simulink model "Demo_veDYNA_cs"  (Simulink 7.6)
settings: Solver=ode1  SolverMode=SingleTasking  StartTime=0  StopTime=15  FixedStep=1/500  RelTol=1e-3
PreLoadFcn:
  | PreScanveDYNAPreLoadFcn(bdroot);
  | check_NUTS_defined;
  | 
  | assignin('base',['model_closed_' bdroot],false);
PostLoadFcn:
  | PreScanveDYNAPostLoadFcn(bdroot);
  | 
InitFcn:
  | vdy_SetExternalInputSource('ManLongCtrl',1,'Brake','other');
  | vdy_SetExternalInputSource('ManLongCtrl',1,'EngineTorque','other');
  | vdy_SetExternalInputSource('ManLatCtrl',1,'Steering','other');
  | 
  | PreScanveDYNAInitFcn(bdroot);
  | PreScanExperimentInitFcn(bdroot)
StopFcn:
  | PreScanExperimentStopFcn(bdroot)
undefined symbols (not defined in the file): at_period, CPT, DiscIntNeverNeededParam, vm_at_pulsewidth, vm_driver_dflt_gain, x_ini_VRML, y_ini_VRML, z_ini_VRML
libraries: dyna_cpt_lib x93, PreScanSimulinkLibrary x10, PreScanUsefulBlocks x4, simulink x4, anilib x3, dyna_lib x3, simulink_extras x2, dyna_manctrl_lib x2, dyna_road_lib x2, dyna_io_lib x1, dyna_demo_lib x1, dyna_usr_maneuver_states_lib x1
(part 4 of 8)

== system Demo_veDYNA_cs/Mazda_RX8_1/AIR_1_Demux/Signal2ArrayOfSignals5 ==
  note: Set mask parameter VECTORLENGTH
      |  to MAXMESSAGES
  note: Initial state of Previous vector block
      | set to zeros(VECTORLENGTH,1)
  LoopIndex : Inport
  Element : Inport  Port=2
  Assignment : Assignment  IndexOptions=Index vector (port)  Indices=1  OutputSizes=1
  Previous vector : Memory  X0=zeros(VECTORLENGTH,1)  InheritSampleTime=on
  ArrayofElements : Outport
  wires:
  Element/1 -> Assignment/2
  LoopIndex/1 -> Assignment/3
  Previous vector/1 -> Assignment/1
  Assignment/1 -> ArrayofElements/1, Previous vector/1

== system Demo_veDYNA_cs/Mazda_RX8_1/AIR_1_Demux/Signal2ArrayOfSignals6 ==
  note: Set mask parameter VECTORLENGTH
      |  to MAXMESSAGES
  note: Initial state of Previous vector block
      | set to zeros(VECTORLENGTH,1)
  LoopIndex : Inport
  Element : Inport  Port=2
  Assignment : Assignment  IndexOptions=Index vector (port)  Indices=1  OutputSizes=1
  Previous vector : Memory  X0=zeros(VECTORLENGTH,1)  InheritSampleTime=on
  ArrayofElements : Outport
  wires:
  Element/1 -> Assignment/2
  LoopIndex/1 -> Assignment/3
  Previous vector/1 -> Assignment/1
  Assignment/1 -> ArrayofElements/1, Previous vector/1

== system Demo_veDYNA_cs/Mazda_RX8_1/SELF_Demux/compas converter ==
  rotz [rad] : Inport
  cart2compas : Subsystem
  rad2deg : Gain  Gain=180/pi
  heading [deg] : Outport
  wires:
  cart2compas/1(heading [deg]) -> heading [deg]/1
  rotz [rad]/1 -> rad2deg/1
  rad2deg/1 -> cart2compas/1(Angle [deg])

== system Demo_veDYNA_cs/Mazda_RX8_1/Simple ACC/Delta control ==
  R : Inport
  theta : Inport  Port=2
  y_dist : Inport  Port=3
  Add : Sum  Inputs=+-
  Complex to Magnitude-Angle1 : ComplexToMagnitudeAngle
  Polar2Cart : Subsystem
  Real-Imag to Complex1 : RealImagToComplex
  Selector : Selector  IndexOptions=Index vector (dialog)  Indices=[1]  OutputSizes=1
  Terminator_1 : Terminator
  delta gain : Gain  Gain=50  SaturateOnIntegerOverflow=on  OutDataTypeStr=Inherit: Same as input  ParamDataTypeStr=Inherit: Same as input
  preview_distance : Constant  Value=2
  delta : Outport
  wires:
  Selector/1 -> Polar2Cart/2(theta)
  theta/1 -> Selector/1
  R/1 -> Polar2Cart/1(R)
  Polar2Cart/1(y) -> Add/1  "yrel"
  Complex to Magnitude-Angle1/1 -> Terminator_1/1
  delta gain/1 -> delta/1
  preview_distance/1 -> Real-Imag to Complex1/1
  Add/1 -> Real-Imag to Complex1/2
  y_dist/1 -> Add/2
  Real-Imag to Complex1/1 -> Complex to Magnitude-Angle1/1
  Complex to Magnitude-Angle1/2 -> delta gain/1

== system Demo_veDYNA_cs/Mazda_RX8_1/Simple ACC/Engine Torque Control ==
  dist Traffic : Inport
  Vehicle Info : Inport  Port=2
  vSoll : Inport  Port=3
  Brake gain : Gain  Gain=60
  Demux Vehicle Info : Subsystem
  Distance Control : Subsystem  TreatAsAtomicUnit=on
  MinMax : MinMax  Inputs=2  SaturateOnIntegerOverflow=on  InputSameDT=on
  Speed Control : Subsystem  TreatAsAtomicUnit=on
  Brake Pedal : Outport
  Engine Torque : Outport  Port=2
  wires:
  Brake gain/1 -> Brake Pedal/1
  Distance Control/2(Brake Pedal) -> Brake gain/1
  Demux Vehicle Info/4(mmot_diff) -> Speed Control/3(mmot_diff)
  Demux Vehicle Info/3(v_akt1) -> Distance Control/3(v_akt)
  vSoll/1 -> Demux Vehicle Info/2(vSoll)
  Demux Vehicle Info/2(mmot_MIN) -> Speed Control/2(mmot_MIN), Distance Control/2(mmot_MIN)
  Demux Vehicle Info/1(mmot_MAX) -> Distance Control/1(mmot_MAX), Speed Control/1(mmot_MAX)
  MinMax/1 -> Engine Torque/1
  Distance Control/1(Engine Torque) -> MinMax/2
  Speed Control/1(Engine Torque) -> MinMax/1
  dist Traffic/1 -> Distance Control/4(s_diff)
  Vehicle Info/1 -> Demux Vehicle Info/1(Vehicle Info)

== system Demo_veDYNA_cs/Nissan_Cabstar_1/SELF_Demux/compas converter ==
  rotz [rad] : Inport
  cart2compas : Subsystem
  rad2deg : Gain  Gain=180/pi
  heading [deg] : Outport
  wires:
  cart2compas/1(heading [deg]) -> heading [deg]/1
  rotz [rad]/1 -> rad2deg/1
  rad2deg/1 -> cart2compas/1(Angle [deg])

== system Demo_veDYNA_cs/Nissan_Cabstar_1/Trajectories/PathFollowerSva_2 ==
  From Workspace : FromWorkspace  VariableName=trajectory  SampleTime=TimeStep  OutputAfterFinalValue=Holding final value
  From Workspace1 : FromWorkspace  VariableName=trajectory  SampleTime=TimeStep  OutputAfterFinalValue=Setting to zero
  Mux : Mux  Inputs=2
  Selector1 : Selector  InputPortWidth=24  IndexOptions=Index vector (dialog)  Indices=[7:18]  OutputSizes=1
  Selector9 : Selector  InputPortWidth=24  IndexOptions=Index vector (dialog)  Indices=[1:6]  OutputSizes=1
  trajectory : Outport
  wires:
  Selector1/1 -> Mux/2
  Selector9/1 -> Mux/1
  Mux/1 -> trajectory/1
  From Workspace1/1 -> Selector1/1
  From Workspace/1 -> Selector9/1

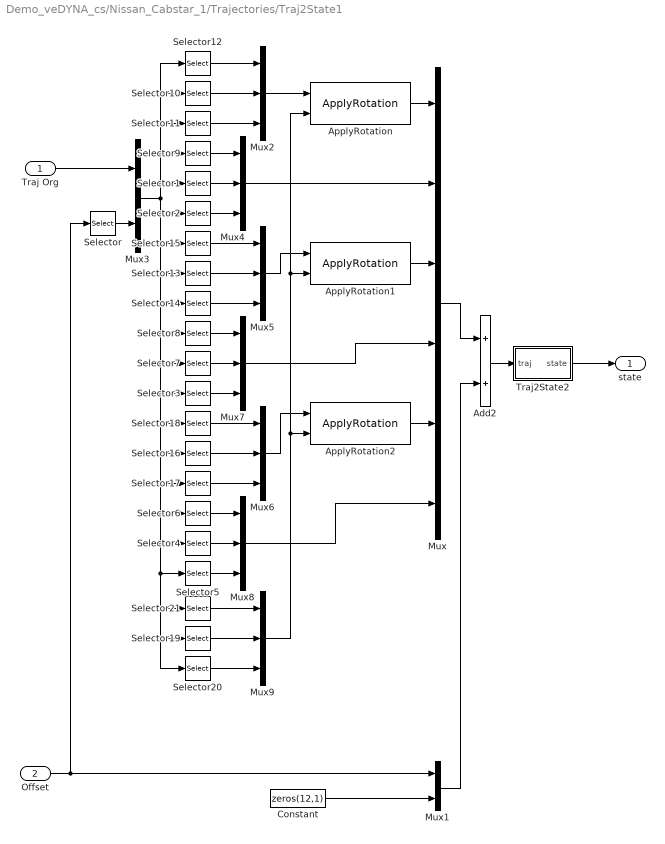
== system Demo_veDYNA_cs/Nissan_Cabstar_1/Trajectories/Traj2State1 ==
  Traj Org : Inport
  Offset : Inport  Port=2
  Add2 : Sum
  ApplyRotation : PreScanSimulinkLibrary/ApplyRotation  SystemSampleTime=-1
  ApplyRotation1 : PreScanSimulinkLibrary/ApplyRotation  SystemSampleTime=-1
  ApplyRotation2 : PreScanSimulinkLibrary/ApplyRotation  SystemSampleTime=-1
  Constant : Constant  Value=zeros(12,1)
  Mux : Mux  Inputs=6
  Mux1 : Mux  Inputs=2
  Mux{2,4..9} (7 alike) : Mux  Inputs=3
  Mux3 : Mux  Inputs=2
  Selector : Selector  InputPortWidth=6  IndexOptions=Index vector (dialog)  Indices=[4 5 6]  OutputSizes=1
  Selector1 : Selector  InputPortWidth=21  IndexOptions=Index vector (dialog)  Indices=[5]  OutputSizes=1
  Selector10 : Selector  InputPortWidth=21  IndexOptions=Index vector (dialog)  Indices=[2]  OutputSizes=1
  Selector11 : Selector  InputPortWidth=21  IndexOptions=Index vector (dialog)  Indices=[3]  OutputSizes=1
  Selector12 : Selector  InputPortWidth=21  IndexOptions=Index vector (dialog)  Indices=[1]  OutputSizes=1
  Selector13 : Selector  InputPortWidth=21  IndexOptions=Index vector (dialog)  Indices=[8]  OutputSizes=1
  Selector14 : Selector  InputPortWidth=21  IndexOptions=Index vector (dialog)  Indices=[9]  OutputSizes=1
  Selector15 : Selector  InputPortWidth=21  IndexOptions=Index vector (dialog)  Indices=[7]  OutputSizes=1
  Selector16 : Selector  InputPortWidth=21  IndexOptions=Index vector (dialog)  Indices=[14]  OutputSizes=1
  Selector17 : Selector  InputPortWidth=21  IndexOptions=Index vector (dialog)  Indices=[15]  OutputSizes=1
  Selector18 : Selector  InputPortWidth=21  IndexOptions=Index vector (dialog)  Indices=[13]  OutputSizes=1
  Selector19 : Selector  InputPortWidth=21  IndexOptions=Index vector (dialog)  Indices=[20]  OutputSizes=1
  Selector2 : Selector  InputPortWidth=21  IndexOptions=Index vector (dialog)  Indices=[6]  OutputSizes=1
  Selector20 : Selector  InputPortWidth=21  IndexOptions=Index vector (dialog)  Indices=[21]  OutputSizes=1
  Selector21 : Selector  InputPortWidth=21  IndexOptions=Index vector (dialog)  Indices=[19]  OutputSizes=1
  Selector3 : Selector  InputPortWidth=21  IndexOptions=Index vector (dialog)  Indices=[12]  OutputSizes=1
  Selector4 : Selector  InputPortWidth=21  IndexOptions=Index vector (dialog)  Indices=[17]  OutputSizes=1
  Selector5 : Selector  InputPortWidth=21  IndexOptions=Index vector (dialog)  Indices=[18]  OutputSizes=1
  Selector6 : Selector  InputPortWidth=21  IndexOptions=Index vector (dialog)  Indices=[16]  OutputSizes=1
  Selector7 : Selector  InputPortWidth=21  IndexOptions=Index vector (dialog)  Indices=[11]  OutputSizes=1
  Selector8 : Selector  InputPortWidth=21  IndexOptions=Index vector (dialog)  Indices=[10]  OutputSizes=1
  Selector9 : Selector  InputPortWidth=21  IndexOptions=Index vector (dialog)  Indices=[4]  OutputSizes=1
  Traj2State2 : Subsystem
  state : Outport
  wires:
  Mux9/1 -> ApplyRotation2/2, ApplyRotation1/2, ApplyRotation/2
  Selector20/1 -> Mux9/3
  Selector19/1 -> Mux9/2
  Selector21/1 -> Mux9/1
  Selector5/1 -> Mux8/3
  Selector4/1 -> Mux8/2
  Selector6/1 -> Mux8/1
  Mux8/1 -> Mux/6
  Mux6/1 -> ApplyRotation2/1
  Mux7/1 -> Mux/4
  ApplyRotation2/1 -> Mux/5
  Selector3/1 -> Mux7/3
  Selector7/1 -> Mux7/2
  Selector8/1 -> Mux7/1
  Mux4/1 -> Mux/2
  Mux5/1 -> ApplyRotation1/1
  ApplyRotation1/1 -> Mux/3
  Mux2/1 -> ApplyRotation/1
  ApplyRotation/1 -> Mux/1
  Selector2/1 -> Mux4/3
  Selector1/1 -> Mux4/2
  Selector9/1 -> Mux4/1
  Selector17/1 -> Mux6/3
  Selector16/1 -> Mux6/2
  Selector18/1 -> Mux6/1
  Selector14/1 -> Mux5/3
  Selector13/1 -> Mux5/2
  Selector15/1 -> Mux5/1
  Selector11/1 -> Mux2/3
  Selector10/1 -> Mux2/2
  Selector12/1 -> Mux2/1
  Mux3/1 -> Selector8/1, Selector7/1, Selector3/1, Selector18/1, Selector16/1, Selector17/1, Selector6/1, Selector20/1, Selector19/1, Selector21/1, Selector5/1, Selector4/1, Selector14/1, Selector13/1, Selector15/1, Selector2/1, Selector1/1, Selector9/1, Selector12/1, Selector10/1, Selector11/1
  Mux1/1 -> Add2/2
  Constant/1 -> Mux1/2
  Add2/1 -> Traj2State2/1(traj)
  Selector/1 -> Mux3/2
  Traj Org/1 -> Mux3/1
  Offset/1 -> Mux1/1, Selector/1
  Mux/1 -> Add2/1
  Traj2State2/1(state) -> state/1

== system Demo_veDYNA_cs/VISUWheels_Mazda_RX8_1/conv_RotWheelFL/RotMat2AxisAngle ==
  RotMat_Visu : Inport
  Data Type Conversion : DataTypeConversion
  Divide : Product  Inputs=*/
  Gain : Gain  Gain=2
  Mux : Mux  Inputs=3
  Mux1 : Mux  Inputs=2
  Saturation1 : Saturate  UpperLimit=3-0.001  LowerLimit=-1+0.001
  Trigonometric Function : Trigonometry
  U1 : Fcn  Expr=u[6]-u[8]
  U2 : Fcn  Expr=u[7]-u[3]
  U3 : Fcn  Expr=u[2]-u[4]
  U_Phi : Fcn  Expr=u[1]+u[5]+u[9]
  U_Phi1 : Fcn  Expr=acos((u(1)-1)/2)
  U_Phi2 : Fcn  Expr=acos((u(1)-1)/2)
  Angles_Visu : Outport
  wires:
  U_Phi2/1 -> Trigonometric Function/1
  Saturation1/1 -> U_Phi2/1
  U_Phi1/1 -> Data Type Conversion/1
  U_Phi/1 -> Saturation1/1, U_Phi1/1
  Divide/1 -> Mux1/1
  Mux1/1 -> Angles_Visu/1
  Gain/1 -> Divide/2
  Mux/1 -> Divide/1
  U3/1 -> Mux/3
  U2/1 -> Mux/2
  U1/1 -> Mux/1
  Trigonometric Function/1 -> Gain/1
  RotMat_Visu/1 -> U_Phi/1, U3/1, U2/1, U1/1
  Data Type Conversion/1 -> Mux1/2

== system Demo_veDYNA_cs/VISUWheels_Mazda_RX8_1/conv_RotWheelFR/RotMat2AxisAngle ==
  RotMat_Visu : Inport
  Data Type Conversion : DataTypeConversion
  Divide : Product  Inputs=*/
  Gain : Gain  Gain=2
  Mux : Mux  Inputs=3
  Mux1 : Mux  Inputs=2
  Saturation1 : Saturate  UpperLimit=3-0.001  LowerLimit=-1+0.001
  Trigonometric Function : Trigonometry
  U1 : Fcn  Expr=u[6]-u[8]
  U2 : Fcn  Expr=u[7]-u[3]
  U3 : Fcn  Expr=u[2]-u[4]
  U_Phi : Fcn  Expr=u[1]+u[5]+u[9]
  U_Phi1 : Fcn  Expr=acos((u(1)-1)/2)
  U_Phi2 : Fcn  Expr=acos((u(1)-1)/2)
  Angles_Visu : Outport
  wires:
  Data Type Conversion/1 -> Mux1/2
  RotMat_Visu/1 -> U1/1, U2/1, U3/1, U_Phi/1
  Trigonometric Function/1 -> Gain/1
  U1/1 -> Mux/1
  U2/1 -> Mux/2
  U3/1 -> Mux/3
  Mux/1 -> Divide/1
  Gain/1 -> Divide/2
  Mux1/1 -> Angles_Visu/1
  Divide/1 -> Mux1/1
  U_Phi/1 -> U_Phi1/1, Saturation1/1
  U_Phi1/1 -> Data Type Conversion/1
  Saturation1/1 -> U_Phi2/1
  U_Phi2/1 -> Trigonometric Function/1

== system Demo_veDYNA_cs/VISUWheels_Mazda_RX8_1/conv_RotWheelRL/RotMat2AxisAngle ==
  RotMat_Visu : Inport
  Data Type Conversion : DataTypeConversion
  Divide : Product  Inputs=*/
  Gain : Gain  Gain=2
  Mux : Mux  Inputs=3
  Mux1 : Mux  Inputs=2
  Saturation1 : Saturate  UpperLimit=3-0.001  LowerLimit=-1+0.001
  Trigonometric Function : Trigonometry
  U1 : Fcn  Expr=u[6]-u[8]
  U2 : Fcn  Expr=u[7]-u[3]
  U3 : Fcn  Expr=u[2]-u[4]
  U_Phi : Fcn  Expr=u[1]+u[5]+u[9]
  U_Phi1 : Fcn  Expr=acos((u(1)-1)/2)
  U_Phi2 : Fcn  Expr=acos((u(1)-1)/2)
  Angles_Visu : Outport
  wires:
  Data Type Conversion/1 -> Mux1/2
  RotMat_Visu/1 -> U1/1, U2/1, U3/1, U_Phi/1
  Trigonometric Function/1 -> Gain/1
  U1/1 -> Mux/1
  U2/1 -> Mux/2
  U3/1 -> Mux/3
  Mux/1 -> Divide/1
  Gain/1 -> Divide/2
  Mux1/1 -> Angles_Visu/1
  Divide/1 -> Mux1/1
  U_Phi/1 -> U_Phi1/1, Saturation1/1
  U_Phi1/1 -> Data Type Conversion/1
  Saturation1/1 -> U_Phi2/1
  U_Phi2/1 -> Trigonometric Function/1

== system Demo_veDYNA_cs/VISUWheels_Mazda_RX8_1/conv_RotWheelRR/RotMat2AxisAngle ==
  RotMat_Visu : Inport
  Data Type Conversion : DataTypeConversion
  Divide : Product  Inputs=*/
  Gain : Gain  Gain=2
  Mux : Mux  Inputs=3
  Mux1 : Mux  Inputs=2
  Saturation1 : Saturate  UpperLimit=3-0.001  LowerLimit=-1+0.001
  Trigonometric Function : Trigonometry
  U1 : Fcn  Expr=u[6]-u[8]
  U2 : Fcn  Expr=u[7]-u[3]
  U3 : Fcn  Expr=u[2]-u[4]
  U_Phi : Fcn  Expr=u[1]+u[5]+u[9]
  U_Phi1 : Fcn  Expr=acos((u(1)-1)/2)
  U_Phi2 : Fcn  Expr=acos((u(1)-1)/2)
  Angles_Visu : Outport
  wires:
  Data Type Conversion/1 -> Mux1/2
  RotMat_Visu/1 -> U1/1, U2/1, U3/1, U_Phi/1
  Trigonometric Function/1 -> Gain/1
  U1/1 -> Mux/1
  U2/1 -> Mux/2
  U3/1 -> Mux/3
  Mux/1 -> Divide/1
  Gain/1 -> Divide/2
  Mux1/1 -> Angles_Visu/1
  Divide/1 -> Mux1/1
  U_Phi/1 -> U_Phi1/1, Saturation1/1
  U_Phi1/1 -> Data Type Conversion/1
  Saturation1/1 -> U_Phi2/1
  U_Phi2/1 -> Trigonometric Function/1

== system Demo_veDYNA_cs/VISUWheels_Mazda_RX8_1/conv_TransWheelFL/pos_ini_Visu ==
  Constant : Constant  Value=x_ini_VRML
  Constant1 : Constant  Value=y_ini_VRML
  Constant2 : Constant  Value=z_ini_VRML
  Mux1 : Mux  Inputs=3
  pos_ini_Visu : Outport
  wires:
  Constant2/1 -> Mux1/3
  Constant1/1 -> Mux1/2
  Mux1/1 -> pos_ini_Visu/1
  Constant/1 -> Mux1/1

== system Demo_veDYNA_cs/VISUWheels_Mazda_RX8_1/conv_TransWheelFL/transISO2Visu ==
  transISO : Inport
  Demux : Demux  Outputs=3
  trans_x_Visu : Outport
  trans_y_Visu : Outport  Port=2
  trans_z_Visu : Outport  Port=3
  wires:
  Demux/3 -> trans_z_Visu/1
  transISO/1 -> Demux/1
  Demux/1 -> trans_x_Visu/1
  Demux/2 -> trans_y_Visu/1  "rot_y"

== system Demo_veDYNA_cs/VISUWheels_Mazda_RX8_1/conv_TransWheelFR/pos_ini_Visu ==
  Constant : Constant  Value=x_ini_VRML
  Constant1 : Constant  Value=y_ini_VRML
  Constant2 : Constant  Value=z_ini_VRML
  Mux1 : Mux  Inputs=3
  pos_ini_Visu : Outport
  wires:
  Constant/1 -> Mux1/1
  Mux1/1 -> pos_ini_Visu/1
  Constant1/1 -> Mux1/2
  Constant2/1 -> Mux1/3

== system Demo_veDYNA_cs/VISUWheels_Mazda_RX8_1/conv_TransWheelFR/transISO2Visu ==
  transISO : Inport
  Demux : Demux  Outputs=3
  trans_x_Visu : Outport
  trans_y_Visu : Outport  Port=2
  trans_z_Visu : Outport  Port=3
  wires:
  Demux/3 -> trans_z_Visu/1
  transISO/1 -> Demux/1
  Demux/1 -> trans_x_Visu/1
  Demux/2 -> trans_y_Visu/1  "rot_y"

== system Demo_veDYNA_cs/VISUWheels_Mazda_RX8_1/conv_TransWheelRL/pos_ini_Visu ==
  Constant : Constant  Value=x_ini_VRML
  Constant1 : Constant  Value=y_ini_VRML
  Constant2 : Constant  Value=z_ini_VRML
  Mux1 : Mux  Inputs=3
  pos_ini_Visu : Outport
  wires:
  Constant/1 -> Mux1/1
  Mux1/1 -> pos_ini_Visu/1
  Constant1/1 -> Mux1/2
  Constant2/1 -> Mux1/3

== system Demo_veDYNA_cs/VISUWheels_Mazda_RX8_1/conv_TransWheelRL/transISO2Visu ==
  transISO : Inport
  Demux : Demux  Outputs=3
  trans_x_Visu : Outport
  trans_y_Visu : Outport  Port=2
  trans_z_Visu : Outport  Port=3
  wires:
  Demux/3 -> trans_z_Visu/1
  transISO/1 -> Demux/1
  Demux/1 -> trans_x_Visu/1
  Demux/2 -> trans_y_Visu/1  "rot_y"

== system Demo_veDYNA_cs/VISUWheels_Mazda_RX8_1/conv_TransWheelRR/pos_ini_Visu ==
  Constant : Constant  Value=x_ini_VRML
  Constant1 : Constant  Value=y_ini_VRML
  Constant2 : Constant  Value=z_ini_VRML
  Mux1 : Mux  Inputs=3
  pos_ini_Visu : Outport
  wires:
  Constant/1 -> Mux1/1
  Mux1/1 -> pos_ini_Visu/1
  Constant1/1 -> Mux1/2
  Constant2/1 -> Mux1/3

== system Demo_veDYNA_cs/VISUWheels_Mazda_RX8_1/conv_TransWheelRR/transISO2Visu ==
  transISO : Inport
  Demux : Demux  Outputs=3
  trans_x_Visu : Outport
  trans_y_Visu : Outport  Port=2
  trans_z_Visu : Outport  Port=3
  wires:
  Demux/3 -> trans_z_Visu/1
  transISO/1 -> Demux/1
  Demux/1 -> trans_x_Visu/1
  Demux/2 -> trans_y_Visu/1  "rot_y"

== system Demo_veDYNA_cs/Vedyna_Vehicle/CPT_IO/IO_DISP ==

== system Demo_veDYNA_cs/Vedyna_Vehicle/CPT_IO/IO_PAR ==

== system Demo_veDYNA_cs/Vedyna_Vehicle/CPT_IO/IO_SW ==

== system Demo_veDYNA_cs/Vedyna_Vehicle/CPT_IO/TA_PAR ==

== system Demo_veDYNA_cs/Vedyna_Vehicle/CPT_IO/mdl_lib4 ==

== system Demo_veDYNA_cs/Vedyna_Vehicle/CPT_MDL/MDL_ANIM ==

== system Demo_veDYNA_cs/Vedyna_Vehicle/CPT_MDL/MDL_PAR ==
  BrkHyd : Subsystem
      mask Display: disp('[Generated]')
  ClutchCtrl : Subsystem
      mask Display: disp('[Generated]')
  Contact : Subsystem
      mask Display: disp('[Generated]')
  Driver : Subsystem
      mask Display: disp('[Generated]')
  Engine : Subsystem
      mask Display: disp('[Generated]')
  GearCtrl : Subsystem
      mask Display: disp('[Generated]')
  ManLatCtrl : Subsystem
      mask Display: disp('[Generated]')
  ManLongCtrl : Subsystem
      mask Display: disp('[Generated]')
  ManSchedule : Subsystem
      mask Display: disp('[Generated]')
  Tmeasy : Subsystem
      mask Display: disp('[Generated]')
  Wheel : Subsystem
      mask Display: disp('[Generated]')

== system Demo_veDYNA_cs/Vedyna_Vehicle/CPT_MDL/MDL_SW ==
  BrkHyd : Subsystem
      mask Display: disp('[Generated]')
  Chassis : Subsystem
      mask Display: disp('[Generated]')
  ClutchCtrl : Subsystem
      mask Display: disp('[Generated]')
  Contact : Subsystem
      mask Display: disp('[Generated]')
  Driveline : Subsystem
      mask Display: disp('[Generated]')
  Driver : Subsystem
      mask Display: disp('[Generated]')
  Engine : Subsystem
      mask Display: disp('[Generated]')
  GearCtrl : Subsystem
      mask Display: disp('[Generated]')
  ManLatCtrl : Subsystem
      mask Display: disp('[Generated]')
  ManLongCtrl : Subsystem
      mask Display: disp('[Generated]')
  ManSchedule : Subsystem
      mask Display: disp('[Generated]')
  Road : Subsystem
      mask Display: disp('[Generated]')
  Simctrl : Subsystem
      mask Display: disp('[Generated]')
  Tmeasy : Subsystem
      mask Display: disp('[Generated]')
  Vehicle : Subsystem
      mask Display: disp('[Generated]')
  Wheel : Subsystem
      mask Display: disp('[Generated]')

== system Demo_veDYNA_cs/Vedyna_Vehicle/CPT_MDL/MDL_TEST ==

== system Demo_veDYNA_cs/Vedyna_Vehicle/CPT_MDL/MDL_USER ==

== system Demo_veDYNA_cs/Vedyna_Vehicle/vdy_mdl/Maneuver Control ==
  note: veDYNA Maneuver Control
  note: COPYRIGHT 2004 by TESIS DYNAware GmbH
  SyncIn : Inport
  Vehicle Info : Inport  Port=2
  Control Factors Adjustment : dyna_demo_lib/Control Factors Adjustment  Description=This module is part of Tesis DYNAware veDYNA.  MaxAccLong=8  MaxDecelLong=-10  ProportionalGain=1.5  IntegralGain=1.5  DerivativeGain=0  ApproxDecelEngFriction=[1 2 3 4 5;-1.2 -0.75 -0.5 -0.35 -0.25]  AccPedalCloseSlewRate=100  AccPedalOpenSlewRate=100  BrakePedalCloseSlewRate=100  BrakePedalOpenSlewRate=100  PedalChangeTime=0.01  BrakePedalDelayTime=0  SteeringWhlAngDelayTime=0  AccPedalDelayTime=0  ClutchPedalDelayTime=0  AccPedalReductionTime=0.25  ReductionTimeBeforeShifting=0.1  AccPedalDuringGearShift=0
  HCI Switch Driver : Subsystem
  HCI Switches : Subsystem
  Maneuver Controller : dyna_manctrl_lib/Maneuver Controller
  Maneuver Controller Inputs : Subsystem
  Maneuver Scheduler : dyna_manctrl_lib/Maneuver Scheduler
  Maneuver Scheduler Inputs : Subsystem
  SyncOut : Outport
  Output to Vehicle : Outport  Port=2
  wires:
  Maneuver Controller/2 -> Control Factors Adjustment/2
  Control Factors Adjustment/2 -> Output to Vehicle/1
  Control Factors Adjustment/1 -> SyncOut/1
  Maneuver Controller/1 -> Control Factors Adjustment/1
  Maneuver Scheduler Inputs/1(Control States) -> Maneuver Scheduler/3
  Maneuver Controller/3 -> Maneuver Scheduler/2
  HCI Switch Driver/1(HCI manCtrl) -> Maneuver Controller/9
  Maneuver Controller Inputs/1("Longitudinal Control Inputs ") -> Maneuver Controller/4
  Maneuver Controller Inputs/2("Lateral Control Inputs ") -> Maneuver Controller/5
  Maneuver Controller Inputs/3("Driver Inputs ") -> Maneuver Controller/6
  Maneuver Controller Inputs/4("Gear Control Inputs ") -> Maneuver Controller/7
  Maneuver Controller Inputs/5("Clutch Control Inputs ") -> Maneuver Controller/8
  Maneuver Scheduler/1 -> Maneuver Controller/1
  Maneuver Scheduler/2 -> Maneuver Controller/2
  HCI Switches/1("HCI Switches ") -> Maneuver Scheduler/4
  Vehicle Info/1 -> Control Factors Adjustment/3, Maneuver Controller/3, Maneuver Scheduler Inputs/1(Vehicle Info)
  SyncIn/1 -> Maneuver Scheduler/1

== system Demo_veDYNA_cs/Vedyna_Vehicle/vdy_mdl/Road ==
  SyncIn : Inport
  veDYNA Road Subsystem : Subsystem  Tag=vedynaRoadMask  mask(vedynaRoadMask){local_comp_inst=1, system_comp_inst=1, cpt_mdl_ini_file=road_ini}
      mask init:
      | vm_comp_mask_cfg('update','Road'); % do not remove
      settings: OpenFcn=vm_comp_mask_cfg('create','Road');
      mask Display: disp('<veDYNA Road>\n\nSystem Instance [1]')
  SyncOut : Outport
  wires:
  SyncIn/1 -> veDYNA Road Subsystem/1(SyncIn)
  veDYNA Road Subsystem/1(SyncOut) -> SyncOut/1

== system Demo_veDYNA_cs/Vedyna_Vehicle/vdy_mdl/Simulation Control ==
  SyncIn : Inport
  veDYNA Simulation Control Subsystem : Subsystem  Tag=vedynaSimctrlMask  mask(vedynaSimctrlMask){local_comp_inst=1, system_comp_inst=1, cpt_mdl_ini_file=simctrl_ini}
      mask init:
      | vm_comp_mask_cfg('update','Simctrl'); % do not remove
      settings: OpenFcn=vm_comp_mask_cfg('create','Simctrl');
      mask Display: disp('<veDYNA Simctrl>\n\nSystem Instance [1]')
  SyncOut : Outport
  wires:
  SyncIn/1 -> veDYNA Simulation Control Subsystem/1(SyncIn)
  veDYNA Simulation Control Subsystem/1(SyncOut) -> SyncOut/1

== system Demo_veDYNA_cs/Vedyna_Vehicle/vdy_mdl/Vehicle System ==
  note: veDYNA Vehicle System
  note: COPYRIGHT 2002 by TESIS DYNAware GmbH
  SyncIn : Inport
  Maneuver Commands : Inport  Port=2
  Input from I/O : Inport  Port=3
  Ground9 : Ground
  Terminator : Terminator
  veDYNA Vehicle Subsystem : Subsystem  Tag=vedynaVehicleMask  mask(vedynaVehicleMask){local_comp_inst=1, system_comp_inst=1, cpt_mdl_ini_file=vehicle_ini}
      mask init:
      | vm_comp_mask_cfg('update','Vehicle'); % do not remove
      settings: OpenFcn=vm_comp_mask_cfg('create','Vehicle');
      mask Display: disp('<veDYNA Vehicle>\n\nSystem Instance [1]')
  SyncOut : Outport
  Output to I/O : Outport  Port=2
  Vehicle Info : Outport  Port=3
  wires:
  Input from I/O/1 -> veDYNA Vehicle Subsystem/3(Input from I/O)
  Ground9/1 -> veDYNA Vehicle Subsystem/4(External Body Forces)
  veDYNA Vehicle Subsystem/3(Reference System) -> Terminator/1
  veDYNA Vehicle Subsystem/1(Output to I/O) -> Output to I/O/1
  Maneuver Commands/1 -> veDYNA Vehicle Subsystem/2(Maneuver Commands)
  SyncIn/1 -> veDYNA Vehicle Subsystem/1(SyncIn)
  veDYNA Vehicle Subsystem/4(SyncOut) -> SyncOut/1
  veDYNA Vehicle Subsystem/2(Vehicle Info) -> Vehicle Info/1

== system Demo_veDYNA_cs/Vedyna_Vehicle/veDYNA2State/Initial Z @ 2 x ts ==
  Z : Inport
  Clock : Clock
      settings: Decimation=10
  Compare To Constant2 : simulink/Logic and Bit Operations/Compare To Constant  SystemSampleTime=-1  relop=<  const=2*str2num(get_param(bdroot,'FixedStep'))  LogicOutDataTypeMode=uint8  ZeroCross=off
  Sum : Sum  Inputs=|+-
  Switch : Switch  Criteria=u2 ~= 0
  Unit Delay : UnitDelay  SampleTime=-1
  Z - Zo : Outport
  wires:
  Switch/1 -> Unit Delay/1, Sum/2
  Unit Delay/1 -> Switch/3
  Clock/1 -> Compare To Constant2/1
  Compare To Constant2/1 -> Switch/2
  Z/1 -> Switch/1, Sum/1
  Sum/1 -> Z - Zo/1

== system Demo_veDYNA_cs/Vedyna_Vehicle/veDYNA2State/Initial Z @ 2 x ts1 ==
  Z : Inport
  Clock : Clock
      settings: Decimation=10
  Compare To Constant2 : simulink/Logic and Bit Operations/Compare To Constant  SystemSampleTime=-1  relop=<  const=2*str2num(get_param(bdroot,'FixedStep'))  LogicOutDataTypeMode=uint8  ZeroCross=off
  Sum : Sum  Inputs=|+-
  Switch : Switch  Criteria=u2 ~= 0
  Unit Delay : UnitDelay  SampleTime=-1
  Z - Zo : Outport
  wires:
  Sum/1 -> Z - Zo/1
  Z/1 -> Sum/1, Switch/1
  Compare To Constant2/1 -> Switch/2
  Clock/1 -> Compare To Constant2/1
  Unit Delay/1 -> Switch/3
  Switch/1 -> Sum/2, Unit Delay/1

== system Demo_veDYNA_cs/BMW_X5_1/SELF_Demux/compas converter/cart2compas ==
  Angle [deg] : Inport
  Constant : Constant  Value=90
  Constant1 : Constant  Value=360
  Gain : Gain  Gain=1/360
  Gain1 : Gain  Gain=360
  Gain2 : Gain  Gain=-1
  Rounding Function : Rounding
  Sum : Sum  Inputs=|-+
  Sum1 : Sum  Inputs=-+|
  Sum2 : Sum  Inputs=++|
  heading [deg] : Outport
  wires:
  Sum2/1 -> heading [deg]/1
  Constant1/1 -> Sum2/1
  Gain2/1 -> Sum2/2
  Constant/1 -> Sum1/1
  Sum1/1 -> Sum/2, Gain/1
  Sum/1 -> Gain2/1
  Angle [deg]/1 -> Sum1/2
  Gain1/1 -> Sum/1
  Rounding Function/1 -> Gain1/1
  Gain/1 -> Rounding Function/1

== system Demo_veDYNA_cs/BMW_X5_1/Trajectories/Traj2State1/Traj2State2 ==
  traj : Inport
  MuxState : Subsystem
  Traj2MuxState_Ext : Subsystem
  state : Outport
  wires:
  Traj2MuxState_Ext/9(Y [rad]) -> MuxState/9(Y [rad])
  Traj2MuxState_Ext/8(P [rad]) -> MuxState/8(P [rad])
  Traj2MuxState_Ext/7(R [rad]) -> MuxState/7(R [rad])
  Traj2MuxState_Ext/6(dz [m/s]) -> MuxState/6(dz [m/s])
  Traj2MuxState_Ext/5(dy [m/s]) -> MuxState/5(dy [m/s])
  Traj2MuxState_Ext/4(dx [m/s]) -> MuxState/4(dx [m/s])
  Traj2MuxState_Ext/3(z [m]) -> MuxState/3(z [m])
  Traj2MuxState_Ext/2(y [m]) -> MuxState/2(y [m])
  Traj2MuxState_Ext/1(x [m]) -> MuxState/1(x [m])
  MuxState/1(state) -> state/1
  traj/1 -> Traj2MuxState_Ext/1(Traj)

== system Demo_veDYNA_cs/Mazda_RX8_1/SELF_Demux/compas converter/cart2compas ==
  Angle [deg] : Inport
  Constant : Constant  Value=90
  Constant1 : Constant  Value=360
  Gain : Gain  Gain=1/360
  Gain1 : Gain  Gain=360
  Gain2 : Gain  Gain=-1
  Rounding Function : Rounding
  Sum : Sum  Inputs=|-+
  Sum1 : Sum  Inputs=-+|
  Sum2 : Sum  Inputs=++|
  heading [deg] : Outport
  wires:
  Sum2/1 -> heading [deg]/1
  Constant1/1 -> Sum2/1
  Gain2/1 -> Sum2/2
  Constant/1 -> Sum1/1
  Sum1/1 -> Sum/2, Gain/1
  Sum/1 -> Gain2/1
  Angle [deg]/1 -> Sum1/2
  Gain1/1 -> Sum/1
  Rounding Function/1 -> Gain1/1
  Gain/1 -> Rounding Function/1

== system Demo_veDYNA_cs/Mazda_RX8_1/Simple ACC/Delta control/Polar2Cart ==
  R : Inport
  theta : Inport  Port=2
  Degrees to Radians : simulink_extras/Transformations/Degrees to Radians  SystemSampleTime=-1
  Fcn1 : Fcn  Expr=sin(-u)
  Product1 : Product  RndMeth=Zero
  y : Outport
  wires:
  theta/1 -> Degrees to Radians/1
  Degrees to Radians/1 -> Fcn1/1
  R/1 -> Product1/1
  Fcn1/1 -> Product1/2
  Product1/1 -> y/1

== system Demo_veDYNA_cs/Mazda_RX8_1/Simple ACC/Engine Torque Control/Demux Vehicle Info ==
  Vehicle Info : Inport
  vSoll : Inport  Port=2
  Bus Selector : BusSelector  OutputSignals=EngineTorqueMax[Nm],EngineTorqueMin[Nm],VehicleSpeed[m|s],TyreRadiusStatFront[m],GearRatioFront[],TyreRadiusStatRear[m],GearRatioRear[],VehicleMass[kg],EngineInertia[kgm2]
  gear_ratio : Subsystem
  mmot diff : Subsystem
  theta_red : Subsystem
  mmot_MAX : Outport
  mmot_MIN : Outport  Port=2
  v_akt1 : Outport  Port=3
  mmot_diff : Outport  Port=4
  wires:
  vSoll/1 -> mmot diff/5(vSoll)
  mmot diff/1(Out1) -> mmot_diff/1
  Bus Selector/2 -> mmot_MIN/1  "<EngineTorqueMin[Nm]>"
  Bus Selector/1 -> mmot_MAX/1  "<EngineTorqueMax[Nm]>"
  Bus Selector/3 -> v_akt1/1, mmot diff/1(vIst)  "<VehicleSpeed[m|s]>"
  theta_red/1(Theta) -> mmot diff/3(Theta)
  gear_ratio/1(GearRatio) -> theta_red/1(gear ratio), mmot diff/2(gear_ratio)
  Vehicle Info/1 -> Bus Selector/1
  Bus Selector/4 -> gear_ratio/1(RStatF)  "<TyreRadiusStatFront[m]>"
  Bus Selector/5 -> gear_ratio/2(GearRatioF)  "<GearRatioFront[]>"
  Bus Selector/6 -> gear_ratio/3(RStatR)  "<TyreRadiusStatRear[m]>"
  Bus Selector/7 -> gear_ratio/4(GearRatioR)  "<GearRatioRear[]>"
  Bus Selector/8 -> theta_red/2(VehMass)  "<VehicleMass[kg]>"
  Bus Selector/9 -> mmot diff/4(Theta Mot)  "<EngineInertia[kgm2]>"

== system Demo_veDYNA_cs/Mazda_RX8_1/Simple ACC/Engine Torque Control/Distance Control ==
  mmot_MAX : Inport
  mmot_MIN : Inport  Port=2
  v_akt : Inport  Port=3
  s_diff : Inport  Port=4
  Constant1 : Constant  Value=0
  Data Type Conversion1 : DataTypeConversion  SaturateOnIntegerOverflow=on  RndMeth=Zero
  Gain3 : Gain  Gain=-.1  SaturateOnIntegerOverflow=on  OutDataTypeStr=Inherit: Same as input  ParamDataTypeStr=Inherit: Same as input
  MinMax1 : MinMax  Function=max  Inputs=2  SaturateOnIntegerOverflow=on  InputSameDT=on
  MinMax2 : MinMax  Inputs=2  SaturateOnIntegerOverflow=on  InputSameDT=on
  P-Controller : Gain  Gain=6
  Product1 : Product  SaturateOnIntegerOverflow=on  InputSameDT=on  OutDataTypeStr=Inherit: Same as first input
  Relational Operator1 : RelationalOperator  Operator=>  InputSameDT=on
  Saturation1 : Saturate  UpperLimit=100  LowerLimit=0
  Sum : Sum  Inputs=|+-  SaturateOnIntegerOverflow=on  InputSameDT=on  OutDataTypeStr=Inherit: Same as first input
  dist_ratio : Gain  Gain=1.2  SaturateOnIntegerOverflow=on  OutDataTypeStr=Inherit: Same as input  ParamDataTypeStr=Inherit: Same as input
  Engine Torque : Outport
  Brake Pedal : Outport  Port=2
  wires:
  Saturation1/1 -> Brake Pedal/1
  Product1/1 -> Saturation1/1
  Gain3/1 -> Product1/2
  Data Type Conversion1/1 -> Product1/1
  Relational Operator1/1 -> Data Type Conversion1/1
  Constant1/1 -> Relational Operator1/1
  P-Controller/1 -> Gain3/1, Relational Operator1/2, MinMax1/1
  MinMax2/1 -> Engine Torque/1
  MinMax1/1 -> MinMax2/2
  mmot_MAX/1 -> MinMax2/1
  mmot_MIN/1 -> MinMax1/2
  dist_ratio/1 -> Sum/2
  Sum/1 -> P-Controller/1
  v_akt/1 -> dist_ratio/1
  s_diff/1 -> Sum/1

== system Demo_veDYNA_cs/Mazda_RX8_1/Simple ACC/Engine Torque Control/Speed Control ==
  mmot_MAX : Inport
  mmot_MIN : Inport  Port=2
  mmot_diff : Inport  Port=3
  MinMax : MinMax  Function=max  Inputs=2  SaturateOnIntegerOverflow=on  InputSameDT=on
  MinMax1 : MinMax  Inputs=2  SaturateOnIntegerOverflow=on  InputSameDT=on
  P-Controller : Gain  Gain=6
  Engine Torque : Outport
  wires:
  mmot_MIN/1 -> MinMax/2
  mmot_MAX/1 -> MinMax1/1
  MinMax1/1 -> Engine Torque/1
  MinMax/1 -> MinMax1/2
  P-Controller/1 -> MinMax/1
  mmot_diff/1 -> P-Controller/1

== system Demo_veDYNA_cs/Nissan_Cabstar_1/SELF_Demux/compas converter/cart2compas ==
  Angle [deg] : Inport
  Constant : Constant  Value=90
  Constant1 : Constant  Value=360
  Gain : Gain  Gain=1/360
  Gain1 : Gain  Gain=360
  Gain2 : Gain  Gain=-1
  Rounding Function : Rounding
  Sum : Sum  Inputs=|-+
  Sum1 : Sum  Inputs=-+|
  Sum2 : Sum  Inputs=++|
  heading [deg] : Outport
  wires:
  Sum2/1 -> heading [deg]/1
  Constant1/1 -> Sum2/1
  Gain2/1 -> Sum2/2
  Constant/1 -> Sum1/1
  Sum1/1 -> Sum/2, Gain/1
  Sum/1 -> Gain2/1
  Angle [deg]/1 -> Sum1/2
  Gain1/1 -> Sum/1
  Rounding Function/1 -> Gain1/1
  Gain/1 -> Rounding Function/1

== system Demo_veDYNA_cs/Nissan_Cabstar_1/Trajectories/Traj2State1/Traj2State2 ==
  traj : Inport
  MuxState : Subsystem
  Traj2MuxState_Ext : Subsystem
  state : Outport
  wires:
  Traj2MuxState_Ext/9(Y [rad]) -> MuxState/9(Y [rad])
  Traj2MuxState_Ext/8(P [rad]) -> MuxState/8(P [rad])
  Traj2MuxState_Ext/7(R [rad]) -> MuxState/7(R [rad])
  Traj2MuxState_Ext/6(dz [m/s]) -> MuxState/6(dz [m/s])
  Traj2MuxState_Ext/5(dy [m/s]) -> MuxState/5(dy [m/s])
  Traj2MuxState_Ext/4(dx [m/s]) -> MuxState/4(dx [m/s])
  Traj2MuxState_Ext/3(z [m]) -> MuxState/3(z [m])
  Traj2MuxState_Ext/2(y [m]) -> MuxState/2(y [m])
  Traj2MuxState_Ext/1(x [m]) -> MuxState/1(x [m])
  MuxState/1(state) -> state/1
  traj/1 -> Traj2MuxState_Ext/1(Traj)

== system Demo_veDYNA_cs/Vedyna_Vehicle/CPT_MDL/MDL_PAR/BrkHyd ==
  System Instance 1 : Subsystem
      mask Display: disp('[Generated]')

== system Demo_veDYNA_cs/Vedyna_Vehicle/CPT_MDL/MDL_PAR/ClutchCtrl ==
  System Instance 1 : Subsystem
      mask Display: disp('[Generated]')

== system Demo_veDYNA_cs/Vedyna_Vehicle/CPT_MDL/MDL_PAR/Contact ==
  System Instance 1 : Subsystem
      mask Display: disp('[Generated]')
  System Instance 2 : Subsystem
      mask Display: disp('[Generated]')
  System Instance 3 : Subsystem
      mask Display: disp('[Generated]')
  System Instance 4 : Subsystem
      mask Display: disp('[Generated]')
  System Instance 5 : Subsystem
      mask Display: disp('[Generated]')
  System Instance 6 : Subsystem
      mask Display: disp('[Generated]')
  System Instance 7 : Subsystem
      mask Display: disp('[Generated]')
  System Instance 8 : Subsystem
      mask Display: disp('[Generated]')

== system Demo_veDYNA_cs/Vedyna_Vehicle/CPT_MDL/MDL_PAR/Driver ==
  System Instance 1 : Subsystem
      mask Display: disp('[Generated]')

== system Demo_veDYNA_cs/Vedyna_Vehicle/CPT_MDL/MDL_PAR/Engine ==
  System Instance 1 : Subsystem
      mask Display: disp('[Generated]')

== system Demo_veDYNA_cs/Vedyna_Vehicle/CPT_MDL/MDL_PAR/GearCtrl ==
  System Instance 1 : Subsystem
      mask Display: disp('[Generated]')

== system Demo_veDYNA_cs/Vedyna_Vehicle/CPT_MDL/MDL_PAR/ManLatCtrl ==
  System Instance 1 : Subsystem
      mask Display: disp('[Generated]')

== system Demo_veDYNA_cs/Vedyna_Vehicle/CPT_MDL/MDL_PAR/ManLongCtrl ==
  System Instance 1 : Subsystem
      mask Display: disp('[Generated]')

== system Demo_veDYNA_cs/Vedyna_Vehicle/CPT_MDL/MDL_PAR/ManSchedule ==

== system Demo_veDYNA_cs/Vedyna_Vehicle/CPT_MDL/MDL_PAR/Tmeasy ==
  System Instance 1 : Subsystem
      mask Display: disp('[Generated]')
  System Instance 2 : Subsystem
      mask Display: disp('[Generated]')
  System Instance 3 : Subsystem
      mask Display: disp('[Generated]')
  System Instance 4 : Subsystem
      mask Display: disp('[Generated]')
  System Instance 5 : Subsystem
      mask Display: disp('[Generated]')
  System Instance 6 : Subsystem
      mask Display: disp('[Generated]')
  System Instance 7 : Subsystem
      mask Display: disp('[Generated]')
  System Instance 8 : Subsystem
      mask Display: disp('[Generated]')

== system Demo_veDYNA_cs/Vedyna_Vehicle/CPT_MDL/MDL_PAR/Wheel ==
  System Instance 1 : Subsystem
      mask Display: disp('[Generated]')
  System Instance 2 : Subsystem
      mask Display: disp('[Generated]')
  System Instance 3 : Subsystem
      mask Display: disp('[Generated]')
  System Instance 4 : Subsystem
      mask Display: disp('[Generated]')
  System Instance 5 : Subsystem
      mask Display: disp('[Generated]')
  System Instance 6 : Subsystem
      mask Display: disp('[Generated]')
  System Instance 7 : Subsystem
      mask Display: disp('[Generated]')
  System Instance 8 : Subsystem
      mask Display: disp('[Generated]')

== system Demo_veDYNA_cs/Vedyna_Vehicle/CPT_MDL/MDL_SW/BrkHyd ==
  System Instance 1 : Subsystem
      mask Display: disp('[Generated]')

== system Demo_veDYNA_cs/Vedyna_Vehicle/CPT_MDL/MDL_SW/Chassis ==
  System Instance 1 : Subsystem
      mask Display: disp('[Generated]')

== system Demo_veDYNA_cs/Vedyna_Vehicle/CPT_MDL/MDL_SW/ClutchCtrl ==
  System Instance 1 : Subsystem
      mask Display: disp('[Generated]')

== system Demo_veDYNA_cs/Vedyna_Vehicle/CPT_MDL/MDL_SW/Contact ==
  System Instance 1 : Subsystem
      mask Display: disp('[Generated]')
  System Instance 2 : Subsystem
      mask Display: disp('[Generated]')
  System Instance 3 : Subsystem
      mask Display: disp('[Generated]')
  System Instance 4 : Subsystem
      mask Display: disp('[Generated]')
  System Instance 5 : Subsystem
      mask Display: disp('[Generated]')
  System Instance 6 : Subsystem
      mask Display: disp('[Generated]')
  System Instance 7 : Subsystem
      mask Display: disp('[Generated]')
  System Instance 8 : Subsystem
      mask Display: disp('[Generated]')

== system Demo_veDYNA_cs/Vedyna_Vehicle/CPT_MDL/MDL_SW/Driveline ==
  System Instance 1 : Subsystem
      mask Display: disp('[Generated]')

== system Demo_veDYNA_cs/Vedyna_Vehicle/CPT_MDL/MDL_SW/Driver ==
  System Instance 1 : Subsystem
      mask Display: disp('[Generated]')

== system Demo_veDYNA_cs/Vedyna_Vehicle/CPT_MDL/MDL_SW/Engine ==
  System Instance 1 : Subsystem
      mask Display: disp('[Generated]')

== system Demo_veDYNA_cs/Vedyna_Vehicle/CPT_MDL/MDL_SW/GearCtrl ==
  System Instance 1 : Subsystem
      mask Display: disp('[Generated]')

== system Demo_veDYNA_cs/Vedyna_Vehicle/CPT_MDL/MDL_SW/ManLatCtrl ==
  System Instance 1 : Subsystem
      mask Display: disp('[Generated]')

== system Demo_veDYNA_cs/Vedyna_Vehicle/CPT_MDL/MDL_SW/ManLongCtrl ==
  System Instance 1 : Subsystem
      mask Display: disp('[Generated]')

== system Demo_veDYNA_cs/Vedyna_Vehicle/CPT_MDL/MDL_SW/ManSchedule ==
  System Instance 1 : Subsystem
      mask Display: disp('[Generated]')
  System Instance 2 : Subsystem
      mask Display: disp('[Generated]')
  System Instance 3 : Subsystem
      mask Display: disp('[Generated]')

== system Demo_veDYNA_cs/Vedyna_Vehicle/CPT_MDL/MDL_SW/Road ==
  System Instance 1 : Subsystem
      mask Display: disp('[Generated]')

== system Demo_veDYNA_cs/Vedyna_Vehicle/CPT_MDL/MDL_SW/Simctrl ==
  System Instance 1 : Subsystem
      mask Display: disp('[Generated]')

== system Demo_veDYNA_cs/Vedyna_Vehicle/CPT_MDL/MDL_SW/Tmeasy ==
  System Instance 1 : Subsystem
      mask Display: disp('[Generated]')
  System Instance 2 : Subsystem
      mask Display: disp('[Generated]')
  System Instance 3 : Subsystem
      mask Display: disp('[Generated]')
  System Instance 4 : Subsystem
      mask Display: disp('[Generated]')
  System Instance 5 : Subsystem
      mask Display: disp('[Generated]')
  System Instance 6 : Subsystem
      mask Display: disp('[Generated]')
  System Instance 7 : Subsystem
      mask Display: disp('[Generated]')
  System Instance 8 : Subsystem
      mask Display: disp('[Generated]')

== system Demo_veDYNA_cs/Vedyna_Vehicle/CPT_MDL/MDL_SW/Vehicle ==
  System Instance 1 : Subsystem
      mask Display: disp('[Generated]')

== system Demo_veDYNA_cs/Vedyna_Vehicle/CPT_MDL/MDL_SW/Wheel ==
  System Instance 1 : Subsystem
      mask Display: disp('[Generated]')
  System Instance 2 : Subsystem
      mask Display: disp('[Generated]')
  System Instance 3 : Subsystem
      mask Display: disp('[Generated]')
  System Instance 4 : Subsystem
      mask Display: disp('[Generated]')
  System Instance 5 : Subsystem
      mask Display: disp('[Generated]')
  System Instance 6 : Subsystem
      mask Display: disp('[Generated]')
  System Instance 7 : Subsystem
      mask Display: disp('[Generated]')
  System Instance 8 : Subsystem
      mask Display: disp('[Generated]')

== system Demo_veDYNA_cs/Vedyna_Vehicle/vdy_mdl/Maneuver Control/HCI Switch Driver ==
  Mux3 : Mux  Inputs=3
  SW_ClutchCtrl_1_HCI : dyna_cpt_lib/CPT_MDL_HCI_SW_ACCESS  Tag=vedynaCPT_MDL_HCI_SW_ACCESS  component=ClutchCtrl  system_inst=1  parameter=HCI
  SW_Driver_1_HCI : dyna_cpt_lib/CPT_MDL_HCI_SW_ACCESS  Tag=vedynaCPT_MDL_HCI_SW_ACCESS  component=Driver  system_inst=1  parameter=HCI
  SW_GearCtrl_1_HCI : dyna_cpt_lib/CPT_MDL_HCI_SW_ACCESS  Tag=vedynaCPT_MDL_HCI_SW_ACCESS  component=GearCtrl  system_inst=1  parameter=HCI
  HCI manCtrl : Outport
  wires:
  Mux3/1 -> HCI manCtrl/1
  SW_ClutchCtrl_1_HCI/1 -> Mux3/3
  SW_GearCtrl_1_HCI/1 -> Mux3/2
  SW_Driver_1_HCI/1 -> Mux3/1

== system Demo_veDYNA_cs/Vedyna_Vehicle/vdy_mdl/Maneuver Control/HCI Switches ==
  Mux : Mux  Inputs=3
  SW_ManSchedule_1_HCI : dyna_cpt_lib/CPT_MDL_HCI_SW_ACCESS  Tag=vedynaCPT_MDL_HCI_SW_ACCESS  component=ManSchedule  system_inst=1  parameter=HCI
  SW_ManSchedule_2_HCI : dyna_cpt_lib/CPT_MDL_HCI_SW_ACCESS  Tag=vedynaCPT_MDL_HCI_SW_ACCESS  component=ManSchedule  system_inst=2  parameter=HCI
  SW_ManSchedule_3_HCI : dyna_cpt_lib/CPT_MDL_HCI_SW_ACCESS  Tag=vedynaCPT_MDL_HCI_SW_ACCESS  component=ManSchedule  system_inst=3  parameter=HCI
  "HCI Switches " : Outport
  wires:
  SW_ManSchedule_3_HCI/1 -> Mux/3
  SW_ManSchedule_2_HCI/1 -> Mux/2
  SW_ManSchedule_1_HCI/1 -> Mux/1
  Mux/1 -> "HCI Switches "/1

== system Demo_veDYNA_cs/Vedyna_Vehicle/vdy_mdl/Maneuver Control/Maneuver Controller Inputs ==
  Clutch Control Inputs : Subsystem
  Driver Inputs : Subsystem
  Gear Control Inputs : Subsystem
  Lateral Control Inputs : Subsystem
  Longitudinal Control Inputs : Subsystem
  "Longitudinal Control Inputs " : Outport
  "Lateral Control Inputs " : Outport  Port=2
  "Driver Inputs " : Outport  Port=3
  "Gear Control Inputs " : Outport  Port=4
  "Clutch Control Inputs " : Outport  Port=5
  wires:
  Driver Inputs/1(Driver Inputs) -> "Driver Inputs "/1
  Gear Control Inputs/1(Gear Control Inputs) -> "Gear Control Inputs "/1
  Clutch Control Inputs/1(Clutch Control Inputs) -> "Clutch Control Inputs "/1
  Lateral Control Inputs/1(Lateral Control Inputs) -> "Lateral Control Inputs "/1
  Longitudinal Control Inputs/1(Longitudinal Control Inputs) -> "Longitudinal Control Inputs "/1

== system Demo_veDYNA_cs/Vedyna_Vehicle/vdy_mdl/Maneuver Control/Maneuver Scheduler Inputs ==
  Vehicle Info : Inport
  Demux : Demux  Outputs=[2,-1]
  Demux1 : Demux  Outputs=[3 1 1 1 1]
  Dot Product : DotProduct  InputSameDT=on  OutDataTypeStr=Inherit: Inherit via internal rule
  Math Functio : Math  Operator=sqrt  SaturateOnIntegerOverflow=on
  Mux1 : Mux  Inputs=3
  Mux2 : Mux  Inputs=6
  Road Information : dyna_road_lib/Road Information  comp_name=Road  RdQueryTyp=xy  nq=1  rd_info_lib=vm_road_info_lib
  Selector4 : Selector  InputPortWidth=21  IndexOptions=Index vector (dialog)  Indices=[1]  OutputSizes=1
  User Definition of Maneuver End States : dyna_usr_maneuver_states_lib/User Definition of Maneuver End States
  m/s_km/h : Gain  Gain=3.6  SaturateOnIntegerOverflow=on  OutDataTypeStr=Inherit: Same as input  ParamDataTypeStr=Inherit: Same as input
  rad_deg : Gain  Gain=180/pi  SaturateOnIntegerOverflow=on  OutDataTypeStr=Inherit: Same as input  ParamDataTypeStr=Inherit: Same as input
  rad_deg1 : Gain  Gain=1e-5  SaturateOnIntegerOverflow=on  OutDataTypeStr=Inherit: Same as input  ParamDataTypeStr=Inherit: Same as input
  rad_deg2 : Gain  Gain=180/pi  SaturateOnIntegerOverflow=on  OutDataTypeStr=Inherit: Same as input  ParamDataTypeStr=Inherit: Same as input
  state_from_vehicleinfo : Selector  IndexOptions=Index vector (dialog)  Indices=[7,8,10,11,12,38,14,66,65]  OutputSizes=1
  Control States : Outport
  wires:
  Demux1/1 -> Dot Product/2, Dot Product/1  "velocity[m/s]"
  Math Functio/1 -> m/s_km/h/1
  Dot Product/1 -> Math Functio/1
  User Definition of Maneuver End States/1 -> Mux2/6
  Mux2/1 -> Mux1/3
  Demux/2 -> Demux1/1
  rad_deg2/1 -> Mux2/5  "[deg/s]"
  rad_deg1/1 -> Mux2/4  "[bar]"
  rad_deg/1 -> Mux2/2  "[deg]"
  m/s_km/h/1 -> Mux2/1  "[km/h]"
  Demux1/5 -> rad_deg2/1  "roll rate [rad/s]"
  Demux1/2 -> rad_deg/1  "steering wheel angle [rad]"
  Demux1/3 -> Mux2/3  "lateral acc.[m/s**2]"
  Demux1/4 -> rad_deg1/1  "brake pressure [Pa]"
  state_from_vehicleinfo/1 -> Demux/1
  Demux/1 -> Road Information/1
  Selector4/1 -> Mux1/2  "distance [m]"
  Mux1/1 -> Control States/1
  [vdy_Simctrl_tsim] -> Mux1/1  "Simulation time [s]"
  Road Information/1 -> Selector4/1
  Vehicle Info/1 -> state_from_vehicleinfo/1

== system Demo_veDYNA_cs/Vedyna_Vehicle/vdy_mdl/Road/veDYNA Road Subsystem ==
  note: veDYNA Road Subsystem
  note: COPYRIGHT 2002 by TESIS DYNAware GmbH
  SyncIn : Inport
  HCI Switch : Subsystem
  veDYNA Road : dyna_road_lib/veDYNA Road
  SyncOut : Outport
  wires:
  HCI Switch/1(HCI Switch) -> veDYNA Road/2
  veDYNA Road/1 -> SyncOut/1
  SyncIn/1 -> veDYNA Road/1

== system Demo_veDYNA_cs/Vedyna_Vehicle/vdy_mdl/Simulation Control/veDYNA Simulation Control Subsystem ==
  note: veDYNA Simulation Control Subsystem
  note: COPYRIGHT 2002 by TESIS DYNAware GmbH
  SyncIn : Inport
  SW_Simctrl_1_Reset : dyna_cpt_lib/CPT_MDL_SW_ACCESS  Tag=vedynaCPT_MDL_HCI_ACCESS  component=Simctrl  system_inst=1  parameter=Reset
  veDYNA Simulation Control : dyna_simctrl_lib/veDYNA Simulation Control  Tag=vedynaSimctrlMask
  SyncOut : Outport
  wires:
  SW_Simctrl_1_Reset/1 -> veDYNA Simulation Control/2
  veDYNA Simulation Control/1 -> SyncOut/1
  SyncIn/1 -> veDYNA Simulation Control/1

== system Demo_veDYNA_cs/Vedyna_Vehicle/vdy_mdl/Vehicle System/veDYNA Vehicle Subsystem ==
  note: veDYNA Vehicle Subsystem
  note: COPYRIGHT 2002 by TESIS DYNAware GmbH
  SyncIn : Inport
  Maneuver Commands : Inport  Port=2
  Input from I/O : Inport  Port=3
  External Body Forces : Inport  Port=4
  Brake System : Subsystem
  External Vehicle Inputs (from I/O) : Subsystem
  HCI Switches : Subsystem
  Maneuver Commands Splitter : Subsystem
  Mux : Mux  Inputs=2
  Selector : Selector  InputPortWidth=32  IndexOptions=Index vector (dialog)  Indices=[1:4]  OutputSizes=1
  Selector1 : Selector  InputPortWidth=32  IndexOptions=Index vector (dialog)  Indices=[5:18]  OutputSizes=1
  Vehicle Outputs to I/O : Subsystem
  veDYNA Vehicle : dyna_vehicle_lib/veDYNA Vehicle
  Output to I/O : Outport
  Vehicle Info : Outport  Port=2
  Reference System : Outport  Port=3
  SyncOut : Outport  Port=4
  wires:
  HCI Switches/1(HCI Switches) -> veDYNA Vehicle/7
  Selector1/1 -> Brake System/2(I/O Vector)
  Selector/1 -> External Vehicle Inputs (from I/O)/2(I/O Vector)
  Input from I/O/1 -> Selector/1, Selector1/1
  Mux/1 -> Vehicle Info/1
  Vehicle Outputs to I/O/2(SyncOut) -> SyncOut/1
  Vehicle Outputs to I/O/1(Output to IO) -> Output to I/O/1
  veDYNA Vehicle/3 -> Vehicle Outputs to I/O/1(SyncIn)
  External Vehicle Inputs (from I/O)/2(External Inputs) -> veDYNA Vehicle/5
  External Body Forces/1 -> veDYNA Vehicle/6
  External Vehicle Inputs (from I/O)/1(SyncOut) -> Brake System/1(SyncIn)
  veDYNA Vehicle/1 -> Mux/2
  Brake System/1(Brake Hydraulics Info) -> Mux/1
  Brake System/2(SyncOut) -> veDYNA Vehicle/1
  Brake System/3(Master Cylinder Pressure) -> veDYNA Vehicle/2
  Brake System/4(Wheel Cylinder Pressures) -> veDYNA Vehicle/3
  veDYNA Vehicle/2 -> Reference System/1
  Maneuver Commands Splitter/4(Maneuver Commands to Vehicle) -> veDYNA Vehicle/4
  Maneuver Commands/1 -> Maneuver Commands Splitter/2(Maneuver Commands)
  SyncIn/1 -> Maneuver Commands Splitter/1(SyncIn)
  Maneuver Commands Splitter/3(Maneuver Commands to Brake System) -> Brake System/3(Brake Pedal Position)
  Maneuver Commands Splitter/2(Maneuver Commands to External Inputs) -> External Vehicle Inputs (from I/O)/3(Maneuver Commands)
  Maneuver Commands Splitter/1(SyncOut) -> External Vehicle Inputs (from I/O)/1(SyncIn)

== system Demo_veDYNA_cs/BMW_X5_1/Trajectories/Traj2State1/Traj2State2/MuxState ==
  x [m] : Inport
  y [m] : Inport  Port=2
  z [m] : Inport  Port=3
  dx [m/s] : Inport  Port=4
  dy [m/s] : Inport  Port=5
  dz [m/s] : Inport  Port=6
  R [rad] : Inport  Port=7
  P [rad] : Inport  Port=8
  Y [rad] : Inport  Port=9
  Mux : Mux  Inputs=9
  state : Outport
  wires:
  z [m]/1 -> Mux/3
  y [m]/1 -> Mux/2
  x [m]/1 -> Mux/1
  Y [rad]/1 -> Mux/9
  P [rad]/1 -> Mux/8
  R [rad]/1 -> Mux/7
  dz [m/s]/1 -> Mux/6
  dy [m/s]/1 -> Mux/5
  dx [m/s]/1 -> Mux/4
  Mux/1 -> state/1

== system Demo_veDYNA_cs/BMW_X5_1/Trajectories/Traj2State1/Traj2State2/Traj2MuxState_Ext ==
  Traj : Inport
  Terminator{1..9} (9 alike) : Terminator
  demux : Subsystem
  x [m] : Outport
  y [m] : Outport  Port=2
  z [m] : Outport  Port=3
  dx [m/s] : Outport  Port=4
  dy [m/s] : Outport  Port=5
  dz [m/s] : Outport  Port=6
  R [rad] : Outport  Port=7
  P [rad] : Outport  Port=8
  Y [rad] : Outport  Port=9
  wires:
  demux/9(Y) -> Y [rad]/1
  demux/7(R) -> R [rad]/1
  demux/5(vely) -> dy [m/s]/1
  demux/4(velx) -> dx [m/s]/1
  demux/10(velR) -> Terminator4/1
  demux/11(velP) -> Terminator5/1
  demux/12(velY) -> Terminator1/1
  demux/13(accx) -> Terminator8/1
  demux/14(accy) -> Terminator9/1
  demux/15(accz) -> Terminator7/1
  demux/18(accY) -> Terminator2/1
  demux/16(accR) -> Terminator3/1
  demux/17(accP) -> Terminator6/1
  demux/3(z) -> z [m]/1
  Traj/1 -> demux/1(traj)
  demux/6(velz) -> dz [m/s]/1
  demux/1(x) -> x [m]/1
  demux/2(y) -> y [m]/1
  demux/8(P) -> P [rad]/1
